simulink model "ASW_OBD"  (R2023a)
settings: configuration reference "cfg_FastTaskCodeGeneration_v01" (kept outside this file)
undefined symbols (not defined in the file): Cdbl_tiSlwTaskSmpTi
(part 2 of 2)

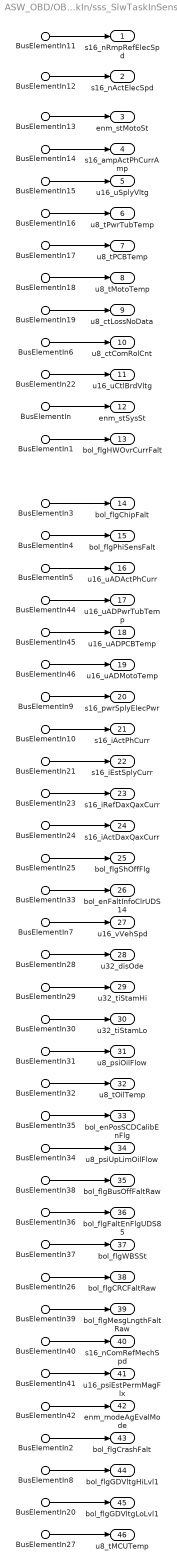
== system ASW_OBD/OBD_SlwTask/vrs_SlwTaskIn/sss_SlwTaskInSens ==
  BusElementIn11 : Inport  PortName=busOBD_SlwTaskIn  Element=s16_nRmpRefElecSpd
  BusElementIn12 : Inport  PortName=busOBD_SlwTaskIn  Element=s16_nActElecSpd
  BusElementIn13 : Inport  PortName=busOBD_SlwTaskIn  Element=enm_stMotoSt
  BusElementIn14 : Inport  PortName=busOBD_SlwTaskIn  Element=s16_ampActPhCurrAmp
  BusElementIn15 : Inport  PortName=busOBD_SlwTaskIn  Element=u16_uSplyVltg
  BusElementIn16 : Inport  PortName=busOBD_SlwTaskIn  Element=u8_tPwrTubTemp
  BusElementIn17 : Inport  PortName=busOBD_SlwTaskIn  Element=u8_tPCBTemp
  BusElementIn18 : Inport  PortName=busOBD_SlwTaskIn  Element=u8_tMotoTemp
  BusElementIn22 : Inport  PortName=busOBD_SlwTaskIn  Element=u16_uCtlBrdVltg
  BusElementIn : Inport  PortName=busOBD_SlwTaskIn  Element=enm_stSysSt
  BusElementIn1 : Inport  PortName=busOBD_SlwTaskIn  Element=bol_flgHWOvrCurrFalt
  BusElementIn3 : Inport  PortName=busOBD_SlwTaskIn  Element=bol_flgChipFalt
  BusElementIn9 : Inport  PortName=busOBD_SlwTaskIn  Element=s16_pwrSplyElecPwr
  BusElementIn10 : Inport  PortName=busOBD_SlwTaskIn  Element=s16_iActPhCurr
  BusElementIn21 : Inport  PortName=busOBD_SlwTaskIn  Element=s16_iEstSplyCurr
  BusElementIn23 : Inport  PortName=busOBD_SlwTaskIn  Element=s16_iRefDaxQaxCurr
  BusElementIn24 : Inport  PortName=busOBD_SlwTaskIn  Element=s16_iActDaxQaxCurr
  BusElementIn25 : Inport  PortName=busOBD_SlwTaskIn  Element=bol_flgShOffFlg
  BusElementIn28 : Inport  PortName=busOBD_SlwTaskIn  Element=u32_disOde
  BusElementIn29 : Inport  PortName=busOBD_SlwTaskIn  Element=u32_tiStamHi
  BusElementIn30 : Inport  PortName=busOBD_SlwTaskIn  Element=u32_tiStamLo
  BusElementIn31 : Inport  PortName=busOBD_SlwTaskIn  Element=u8_psiOilFlow
  BusElementIn32 : Inport  PortName=busOBD_SlwTaskIn  Element=u8_tOilTemp
  BusElementIn34 : Inport  PortName=busOBD_SlwTaskIn  Element=u8_psiUpLimOilFlow
  BusElementIn35 : Inport  PortName=busOBD_SlwTaskIn  Element=bol_enPosSCDCalibEnFlg
  BusElementIn33 : Inport  PortName=busOBD_SlwTaskIn  Element=bol_enFaltInfoClrUDS14
  BusElementIn36 : Inport  PortName=busOBD_SlwTaskIn  Element=bol_flgFaltEnFlgUDS85
  BusElementIn37 : Inport  PortName=busOBD_SlwTaskIn  Element=bol_flgWBSSt
  BusElementIn38 : Inport  PortName=busOBD_SlwTaskIn  Element=bol_flgBusOffFaltRaw
  BusElementIn19 : Inport  PortName=busOBD_SlwTaskIn  Element=bol_flgComLosFaltRaw
  BusElementIn26 : Inport  PortName=busOBD_SlwTaskIn  Element=bol_flgCRCFaltRaw
  BusElementIn39 : Inport  PortName=busOBD_SlwTaskIn  Element=bol_flgMesgLngthFaltRaw
  BusElementIn40 : Inport  PortName=busOBD_SlwTaskIn  Element=s16_nComRefMechSpd
  BusElementIn41 : Inport  PortName=busOBD_SlwTaskIn  Element=u16_psiEstPermMagFlx
  BusElementIn4 : Inport  PortName=busOBD_SlwTaskIn  Element=bol_flgPhiSensFalt
  BusElementIn42 : Inport  PortName=busOBD_SlwTaskIn  Element=enm_modeAgEvalMode
  BusElementIn44 : Inport  PortName=busOBD_SlwTaskIn  Element=u16_uADPwrTubTemp
  BusElementIn45 : Inport  PortName=busOBD_SlwTaskIn  Element=u16_uADPCBTemp
  BusElementIn46 : Inport  PortName=busOBD_SlwTaskIn  Element=u16_uADMotoTemp
  BusElementIn5 : Inport  PortName=busOBD_SlwTaskIn  Element=u16_uADActPhCurr
  BusElementIn6 : Inport  PortName=busOBD_SlwTaskIn  Element=u8_ctComRolCnt
  BusElementIn7 : Inport  PortName=busOBD_SlwTaskIn  Element=u16_vVehSpd
  BusElementIn2 : Inport  PortName=busOBD_SlwTaskIn  Element=bol_flgCrashFalt
  BusElementIn8 : Inport  PortName=busOBD_SlwTaskIn  Element=bol_flgGDVltgHiLvl1
  BusElementIn20 : Inport  PortName=busOBD_SlwTaskIn  Element=bol_flgGDVltgLoLvl1
  BusElementIn27 : Inport  PortName=busOBD_SlwTaskIn  Element=u8_tMCUTemp
  s16_nRmpRefElecSpd : Outport
  s16_nActElecSpd : Outport  Port=2
  enm_stMotoSt : Outport  Port=3
  s16_ampActPhCurrAmp : Outport  Port=4
  u16_uSplyVltg : Outport  Port=5
  u8_tPwrTubTemp : Outport  Port=6
  u8_tPCBTemp : Outport  Port=7
  u8_tMotoTemp : Outport  Port=8
  u8_ctLossNoData : Outport  Port=9
  u8_ctComRolCnt : Outport  Port=10
  u16_uCtlBrdVltg : Outport  Port=11
  enm_stSysSt : Outport  Port=12
  bol_flgHWOvrCurrFalt : Outport  Port=13
  bol_flgChipFalt : Outport  Port=14
  bol_flgPhiSensFalt : Outport  Port=15
  u16_uADActPhCurr : Outport  Port=16
  u16_uADPwrTubTemp : Outport  Port=17
  u16_uADPCBTemp : Outport  Port=18
  u16_uADMotoTemp : Outport  Port=19
  s16_pwrSplyElecPwr : Outport  Port=20
  s16_iActPhCurr : Outport  Port=21
  s16_iEstSplyCurr : Outport  Port=22
  s16_iRefDaxQaxCurr : Outport  Port=23
  s16_iActDaxQaxCurr : Outport  Port=24
  bol_flgShOffFlg : Outport  Port=25
  bol_enFaltInfoClrUDS14 : Outport  Port=26
  u16_vVehSpd : Outport  Port=27
  u32_disOde : Outport  Port=28
  u32_tiStamHi : Outport  Port=29
  u32_tiStamLo : Outport  Port=30
  u8_psiOilFlow : Outport  Port=31
  u8_tOilTemp : Outport  Port=32
  bol_enPosSCDCalibEnFlg : Outport  Port=33
  u8_psiUpLimOilFlow : Outport  Port=34
  bol_flgBusOffFaltRaw : Outport  Port=35
  bol_flgFaltEnFlgUDS85 : Outport  Port=36
  bol_flgWBSSt : Outport  Port=37
  bol_flgCRCFaltRaw : Outport  Port=38
  bol_flgMesgLngthFaltRaw : Outport  Port=39
  s16_nComRefMechSpd : Outport  Port=40
  u16_psiEstPermMagFlx : Outport  Port=41
  enm_modeAgEvalMode : Outport  Port=42
  bol_flgCrashFalt : Outport  Port=43
  bol_flgGDVltgHiLvl1 : Outport  Port=44
  bol_flgGDVltgLoLvl1 : Outport  Port=45
  u8_tMCUTemp : Outport  Port=46
  wires:
  BusElementIn24/1 -> s16_iActDaxQaxCurr/1
  BusElementIn46/1 -> u16_uADMotoTemp/1
  BusElementIn/1 -> enm_stSysSt/1
  BusElementIn44/1 -> u16_uADPwrTubTemp/1
  BusElementIn16/1 -> u8_tPwrTubTemp/1
  BusElementIn33/1 -> bol_enFaltInfoClrUDS14/1
  BusElementIn12/1 -> s16_nActElecSpd/1
  BusElementIn5/1 -> u16_uADActPhCurr/1
  BusElementIn29/1 -> u32_tiStamHi/1
  BusElementIn42/1 -> enm_modeAgEvalMode/1
  BusElementIn31/1 -> u8_psiOilFlow/1
  BusElementIn26/1 -> bol_flgCRCFaltRaw/1
  BusElementIn20/1 -> bol_flgGDVltgLoLvl1/1
  BusElementIn7/1 -> u16_vVehSpd/1
  BusElementIn28/1 -> u32_disOde/1
  BusElementIn40/1 -> s16_nComRefMechSpd/1
  BusElementIn23/1 -> s16_iRefDaxQaxCurr/1
  BusElementIn27/1 -> u8_tMCUTemp/1
  BusElementIn6/1 -> u8_ctComRolCnt/1
  BusElementIn22/1 -> u16_uCtlBrdVltg/1
  BusElementIn10/1 -> s16_iActPhCurr/1
  BusElementIn38/1 -> bol_flgBusOffFaltRaw/1
  BusElementIn19/1 -> u8_ctLossNoData/1
  BusElementIn30/1 -> u32_tiStamLo/1
  BusElementIn41/1 -> u16_psiEstPermMagFlx/1
  BusElementIn34/1 -> u8_psiUpLimOilFlow/1
  BusElementIn37/1 -> bol_flgWBSSt/1
  BusElementIn39/1 -> bol_flgMesgLngthFaltRaw/1
  BusElementIn45/1 -> u16_uADPCBTemp/1
  BusElementIn8/1 -> bol_flgGDVltgHiLvl1/1
  BusElementIn1/1 -> bol_flgHWOvrCurrFalt/1
  BusElementIn32/1 -> u8_tOilTemp/1
  BusElementIn21/1 -> s16_iEstSplyCurr/1
  BusElementIn36/1 -> bol_flgFaltEnFlgUDS85/1
  BusElementIn35/1 -> bol_enPosSCDCalibEnFlg/1
  BusElementIn18/1 -> u8_tMotoTemp/1
  BusElementIn25/1 -> bol_flgShOffFlg/1
  BusElementIn2/1 -> bol_flgCrashFalt/1
  BusElementIn11/1 -> s16_nRmpRefElecSpd/1
  BusElementIn13/1 -> enm_stMotoSt/1
  BusElementIn14/1 -> s16_ampActPhCurrAmp/1
  BusElementIn15/1 -> u16_uSplyVltg/1
  BusElementIn4/1 -> bol_flgPhiSensFalt/1
  BusElementIn9/1 -> s16_pwrSplyElecPwr/1
  BusElementIn17/1 -> u8_tPCBTemp/1
  BusElementIn3/1 -> bol_flgChipFalt/1

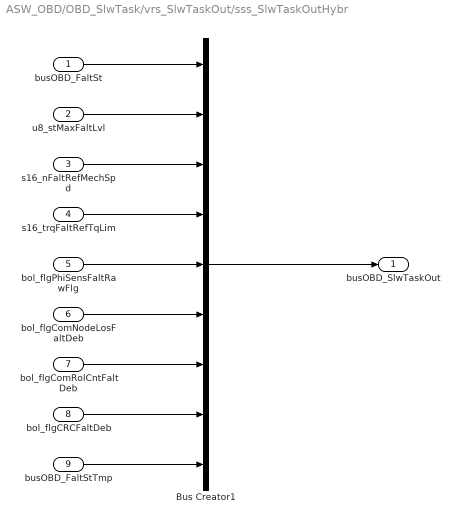
== system ASW_OBD/OBD_SlwTask/vrs_SlwTaskOut/sss_SlwTaskOutHybr ==
  busOBD_FaltSt : Inport
  u8_stMaxFaltLvl : Inport  Port=2
  s16_nFaltRefMechSpd : Inport  Port=3
  s16_trqFaltRefTqLim : Inport  Port=4
  bol_flgPhiSensFaltRawFlg : Inport  Port=5
  bol_flgComNodeLosFaltDeb : Inport  Port=6
  bol_flgComRolCntFaltDeb : Inport  Port=7
  bol_flgCRCFaltDeb : Inport  Port=8
  busOBD_FaltStTmp : Inport  Port=9
  Bus Creator1 : BusCreator  Inputs=9  OutDataTypeStr=Bus: BUS_OBD_SLW_TASK_OUT  NonVirtualBus=on
      settings: InheritFromInputs=off
  busOBD_SlwTaskOut : Outport
  wires:
  busOBD_FaltSt/1 -> Bus Creator1/1
  Bus Creator1/1 -> busOBD_SlwTaskOut/1
  s16_nFaltRefMechSpd/1 -> Bus Creator1/3
  s16_trqFaltRefTqLim/1 -> Bus Creator1/4
  u8_stMaxFaltLvl/1 -> Bus Creator1/2
  bol_flgPhiSensFaltRawFlg/1 -> Bus Creator1/5
  bol_flgComNodeLosFaltDeb/1 -> Bus Creator1/6
  bol_flgComRolCntFaltDeb/1 -> Bus Creator1/7
  bol_flgCRCFaltDeb/1 -> Bus Creator1/8
  busOBD_FaltStTmp/1 -> Bus Creator1/9

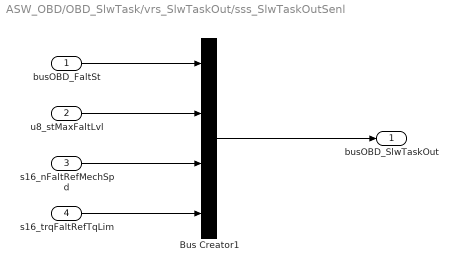
== system ASW_OBD/OBD_SlwTask/vrs_SlwTaskOut/sss_SlwTaskOutSenl ==
  busOBD_FaltSt : Inport
  u8_stMaxFaltLvl : Inport  Port=2
  s16_nFaltRefMechSpd : Inport  Port=3
  s16_trqFaltRefTqLim : Inport  Port=4
  Bus Creator1 : BusCreator  Inputs=4  OutDataTypeStr=Bus: BUS_OBD_SLW_TASK_OUT  NonVirtualBus=on
      settings: InheritFromInputs=off
  busOBD_SlwTaskOut : Outport
  wires:
  s16_trqFaltRefTqLim/1 -> Bus Creator1/4
  Bus Creator1/1 -> busOBD_SlwTaskOut/1
  u8_stMaxFaltLvl/1 -> Bus Creator1/2
  busOBD_FaltSt/1 -> Bus Creator1/1
  s16_nFaltRefMechSpd/1 -> Bus Creator1/3

== system ASW_OBD/OBD_SlwTask/vrs_SlwTaskOut/sss_SlwTaskOutSens ==
  busOBD_FaltSt : Inport
  u8_stMaxFaltLvl : Inport  Port=2
  s16_nFaltRefMechSpd : Inport  Port=3
  s16_trqFaltRefTqLim : Inport  Port=4
  Bus Creator1 : BusCreator  Inputs=4  OutDataTypeStr=Bus: BUS_OBD_SLW_TASK_OUT  NonVirtualBus=on
      settings: InheritFromInputs=off
  busOBD_SlwTaskOut : Outport
  wires:
  Bus Creator1/1 -> busOBD_SlwTaskOut/1
  busOBD_FaltSt/1 -> Bus Creator1/1
  u8_stMaxFaltLvl/1 -> Bus Creator1/2
  s16_nFaltRefMechSpd/1 -> Bus Creator1/3
  s16_trqFaltRefTqLim/1 -> Bus Creator1/4
